simulink model "HomeTaskModel"  (R2022b)
settings: Solver=VariableStepAuto  StartTime=0.0  StopTime=11  RelTol=1e-3
values from neighbouring files (symbols this model uses):
  alpha_filt = 2    [hometask.m]
  x0 = [-0.88 0.46 -6]    [hometask.m]
settings Model: Creator=ilya  LastModifiedBy=ilya

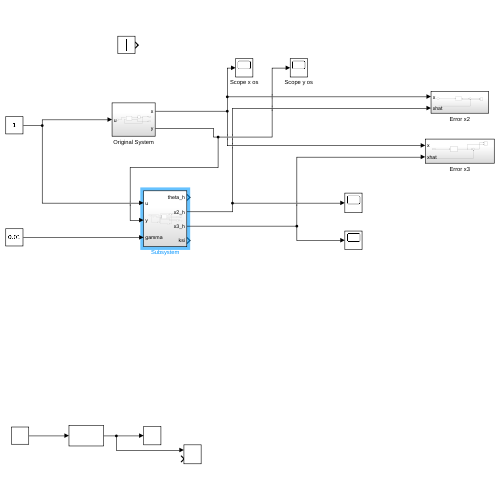
[thumbnail: Simulink's stored preview of the top-level diagram]
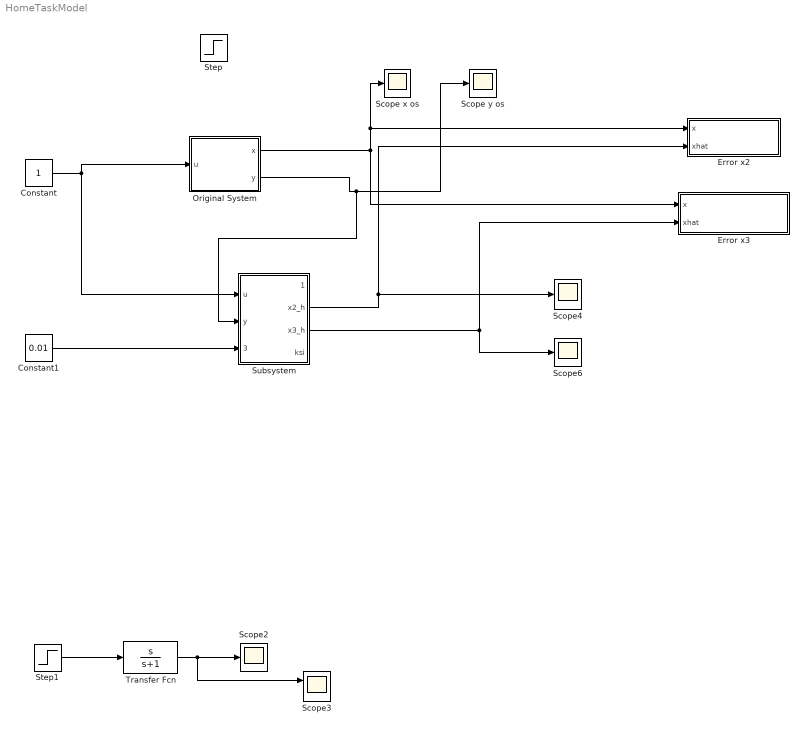
== system HomeTaskModel ==
  Constant : Constant
  Constant1 : Constant  Value=0.01
  Error x2 : Subsystem
  Error x3 : Subsystem
  Original System : Subsystem
  Scope x os : Scope
  Scope y os : Scope
  Scope2 : Scope
  Scope3 : Scope  NumInputPorts=2
  Scope4 : Scope
  Scope6 : Scope
  Step : Step  SampleTime=0
  Step1 : Step  SampleTime=0
  Subsystem : Subsystem
  Transfer Fcn : TransferFcn  Numerator=[1 0]  Denominator=[1 1]
  wires:
  Constant/1 -> Original System/1(u), Subsystem/1(u)
  Transfer Fcn/1 -> Scope3/1, Scope2/1
  Step1/1 -> Transfer Fcn/1
  Subsystem/2(x2_h) -> Scope4/1, Error x2/2(xhat)
  Constant1/1 -> Subsystem/3(gamma)
  Subsystem/3(x3_h) -> Scope6/1, Error x3/2(xhat)
  Original System/2(y) -> Subsystem/2(y), Scope y os/1
  Original System/1(x) -> Error x2/1(x), Scope x os/1, Error x3/1(x)

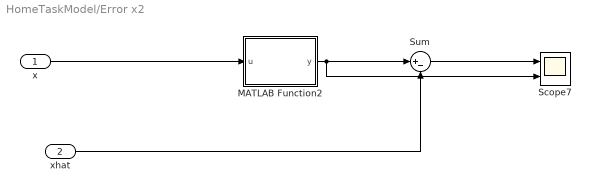
== system HomeTaskModel/Error x2 ==
  x : Inport
  xhat : Inport  Port=2
  MATLAB Function2 : MATLAB Function  TreatAsAtomicUnit=on
  Scope7 : Scope  NumInputPorts=2
  Sum : Sum  Inputs=|+-
  wires:
  xhat/1 -> Sum/2
  Sum/1 -> Scope7/1
  MATLAB Function2/1(y) -> Scope7/2, Sum/1
  x/1 -> MATLAB Function2/1(u)

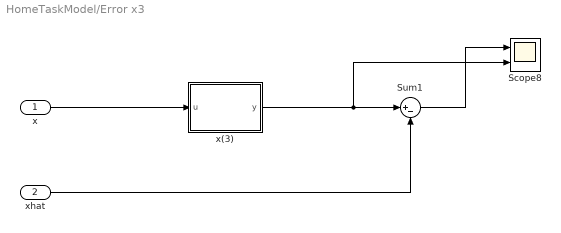
== system HomeTaskModel/Error x3 ==
  x : Inport
  xhat : Inport  Port=2
  Scope8 : Scope  NumInputPorts=2
  Sum1 : Sum  Inputs=|+-
  x(3) : MATLAB Function  TreatAsAtomicUnit=on
  wires:
  Sum1/1 -> Scope8/1
  x(3)/1(y) -> Scope8/2, Sum1/1
  xhat/1 -> Sum1/2
  x/1 -> x(3)/1(u)

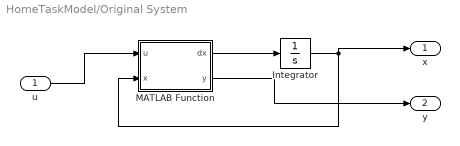
== system HomeTaskModel/Original System ==
  u : Inport
  Integrator : Integrator  InitialCondition=x0
  MATLAB Function : MATLAB Function  TreatAsAtomicUnit=on
  x : Outport
  y : Outport  Port=2
  wires:
  MATLAB Function/1(dx) -> Integrator/1
  MATLAB Function/2(y) -> y/1
  u/1 -> MATLAB Function/1(u)
  Integrator/1 -> MATLAB Function/2(x), x/1

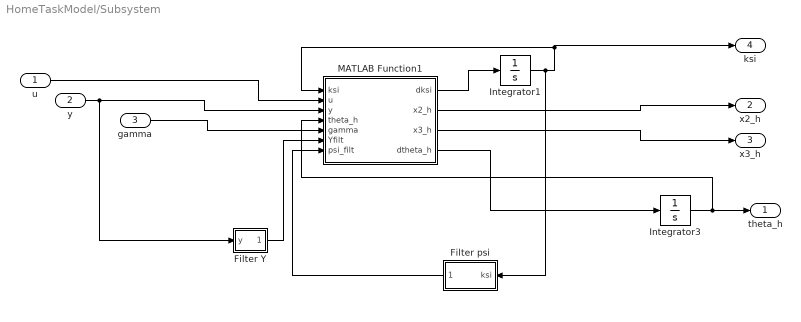
== system HomeTaskModel/Subsystem ==
  u : Inport
  y : Inport  Port=2
  gamma : Inport  Port=3
  Filter Y : Subsystem
  Filter psi : Subsystem
  Integrator1 : Integrator  InitialCondition=[0 0]
  Integrator3 : Integrator  InitialCondition=0.01
  MATLAB Function1 : MATLAB Function  TreatAsAtomicUnit=on
  theta_h : Outport
  x2_h : Outport  Port=2
  x3_h : Outport  Port=3
  ksi : Outport  Port=4
  wires:
  u/1 -> MATLAB Function1/2(u)
  MATLAB Function1/3(x3_h) -> x3_h/1
  MATLAB Function1/2(x2_h) -> x2_h/1
  MATLAB Function1/1(dksi) -> Integrator1/1
  Integrator1/1 -> Filter psi/1(ksi), ksi/1, MATLAB Function1/1(ksi)
  y/1 -> Filter Y/1(y), MATLAB Function1/3(y)
  gamma/1 -> MATLAB Function1/5(gamma)
  Integrator3/1 -> MATLAB Function1/4(theta_h), theta_h/1
  MATLAB Function1/4(dtheta_h) -> Integrator3/1
  Filter Y/1(Yfilt) -> MATLAB Function1/6(Yfilt)
  Filter psi/1(psi_filt) -> MATLAB Function1/7(psi_filt)

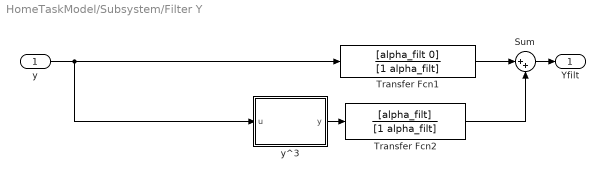
== system HomeTaskModel/Subsystem/Filter Y ==
  y : Inport
  Sum : Sum  Inputs=|++
  Transfer Fcn1 : TransferFcn  Numerator=[alpha_filt 0]  Denominator=[1 alpha_filt]
  Transfer Fcn2 : TransferFcn  Numerator=[alpha_filt]  Denominator=[1 alpha_filt]
  y^3 : MATLAB Function  TreatAsAtomicUnit=on
  Yfilt : Outport
  wires:
  y^3/1(y) -> Transfer Fcn2/1
  Transfer Fcn2/1 -> Sum/2
  Transfer Fcn1/1 -> Sum/1
  Sum/1 -> Yfilt/1
  y/1 -> y^3/1(u), Transfer Fcn1/1

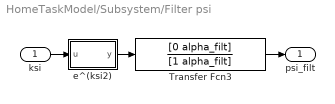
== system HomeTaskModel/Subsystem/Filter psi ==
  ksi : Inport
  Transfer Fcn3 : TransferFcn  Numerator=[0 alpha_filt]  Denominator=[1 alpha_filt]
  e^(ksi2) : MATLAB Function  TreatAsAtomicUnit=on
  psi_filt : Outport
  wires:
  e^(ksi2)/1(y) -> Transfer Fcn3/1
  ksi/1 -> e^(ksi2)/1(u)
  Transfer Fcn3/1 -> psi_filt/1

== matlab function HomeTaskModel/Subsystem/MATLAB Function1 ==
  data: ksi input; u input; dksi output; y input; theta_h input; gamma input; x2_h output; x3_h output; Yfilt input; psi_filt input; dtheta_h output
function [dksi,x2_h, x3_h, dtheta_h] = fcn(ksi, u, y, theta_h, gamma, Yfilt, psi_filt)
    dksi1 = -ksi(1) + y^2 + sin(y);
    dksi2 = u*y + (y^2 + 1)^(-1);
    dtheta_h = gamma * psi_filt * (Yfilt - psi_filt * theta_h);
    x2_h = ksi(1);
    x3_h = ksi(2) + real(log(complex(theta_h)));%log(theta_h);
    dksi = [dksi1, dksi2];

== matlab function HomeTaskModel/Original System/MATLAB Function ==
  data: dx output; u input; y output; x input
function [dx,y] = fcn(u,x)

dx1 = -x(1)^3 + exp(x(3));
dx2 = -x(2) + x(1)^2 + sin(x(1));
dx3 = 1/(x(1)^2 + 1) + x(1) * u;
y = x(1);
dx = [dx1, dx2, dx3];

== matlab function HomeTaskModel/Error x2/MATLAB Function2 ==
  data: u input; y output
function y = fcn(u)

y = u(2);

== matlab function HomeTaskModel/Error x3/x(3) ==
  data: u input; y output
function y = fcn(u)

y = u(3);

== matlab function HomeTaskModel/Subsystem/Filter Y/y^3 ==
  data: u input; y output
function y = fcn(u)

y = u^3;

== matlab function HomeTaskModel/Subsystem/Filter psi/e^(ksi2) ==
  data: u input; y output
function y = fcn(u)

y = exp(u(2));
